simulink model "untitled (2)"  (R2020a)
settings: Solver=VariableStepAuto  StartTime=0.0  StopTime=3  RelTol=1e-3
libraries: simulink x1
settings Model: Creator=nose  LastModifiedBy=nose

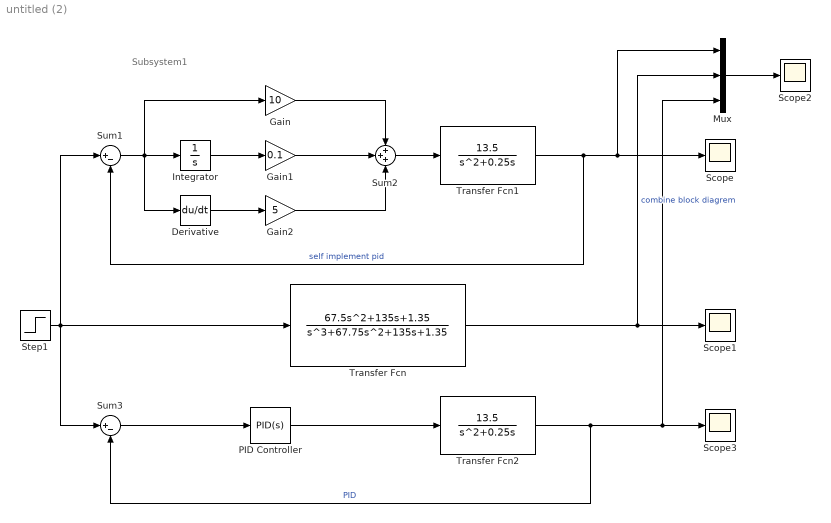
== system untitled (2) ==
  note: Subsystem1
  Derivative : Derivative
  Gain : Gain  Gain=10
  Gain1 : Gain  Gain=0.1
  Gain2 : Gain  Gain=5
  Integrator : Integrator
  Mux : Mux  Inputs=3
  PID Controller : simulink/Continuous/PID Controller  Controller=PID  Form=Parallel  TimeDomain=Continuous-time  UseExternalTs=off  SampleTime=-1  IntegratorMethod=Forward Euler  FilterMethod=Forward Euler  ControllerParametersSource=internal  P=10  I=0.1  D=5  UseFilter=on  N=100  TunerSelectOption=Transfer Function Based (PID Tuner App)  InitialConditionSource=internal  InitialConditionForIntegrator=0  InitialConditionForFilter=0  DifferentiatorICPrevScaledInput=0  ExternalReset=none  TrackingMode=off  Kt=1  LimitOutput=off  UpperSaturationLimit=inf  LowerSaturationLimit=-inf  LinearizeAsGain=on  AntiWindupMode=none  Kb=1  POutMin=[]  POutMax=[]  IOutMin=[]  IOutMax=[]  DOutMin=[]  DOutMax=[]  NOutMin=[]  NOutMax=[]  SumOutMin=[]  SumOutMax=[]  SaturationOutMin=[]  SaturationOutMax=[]  PParamMin=[]  PParamMax=[]  IParamMin=[]  IParamMax=[]  DParamMin=[]  DParamMax=[]  NParamMin=[]  NParamMax=[]  KbParamMin=[]  KbParamMax=[]  KtParamMin=[]  KtParamMax=[]  KbOutMin=[]  KbOutMax=[]  KtOutMin=[]  KtOutMax=[]  IntegratorOutMin=[]  IntegratorOutMax=[]  FilterOutMin=[]  FilterOutMax=[]  SumI1OutMin=[]  SumI1OutMax=[]  SumI2OutMin=[]  SumI2OutMax=[]  SumI3OutMin=[]  SumI3OutMax=[]  SumI4OutMin=[]  SumI4OutMax=[]  SumDOutMin=[]  SumDOutMax=[]  DifferentiatorOutMin=[]  DifferentiatorOutMax=[]  FilterDiffOutCoefMin=[]  FilterDiffOutCoefMax=[]  ReciprocalOutMin=[]  ReciprocalOutMax=[]  SumDenOutMin=[]  SumDenOutMax=[]  SumNumOutMin=[]  SumNumOutMax=[]  DivideOutMin=[]  DivideOutMax=[]  UdiffTsProdOutMin=[]  UdiffTsProdOutMax=[]  NTsProdOutMin=[]  NTsProdOutMax=[]  UintegralTsProdOutMin=[]  UintegralTsProdOutMax=[]  UngainTsProdOutMin=[]  UngainTsProdOutMax=[]  IntegratorContinuousStateAttributes=''  IntegratorStateMustResolveToSignalObject=off  IntegratorRTWStateStorageClass=Auto  FilterContinuousStateAttributes=''  FilterStateMustResolveToSignalObject=off  FilterRTWStateStorageClass=Auto  ParallelPVariant=InternalParameters  IdealPVariant=Disabled  IVariant=InternalParameters  DVariant=InternalParameters  IntegratorVariant=Continuous  SatVariant=Disabled  AWVariant=Passthrough  PCopyVariant=Disabled  TRVariant=Disabled  FdbkBlocksVariant=Forward  IdealPFdbkVariant=Disabled  SatFdbkVariant=Disabled  DerivativeFilterVariant=ContFilter  NVariant=InternalParameters  NCopyVariant=Disabled  FilterICVariant=InternalICsFilter  IntegratorICVariant=InternalICs  ExternalResetVariant=Disabled  TRSumVariant=Passthrough  SumFdbkVariant=Disabled  SumVariant=Sum_PID  TsampFilterVariant=InternalTs  TsampNgainVariant=Passthrough  TsampIntegralVariant=Passthrough
  Scope{,1..3} (4 alike) : Scope
  Step1 : Step  SampleTime=0  ZeroCross=off
  Sum1 : Sum  Inputs=|+-
  Sum2 : Sum  Inputs=+++
  Sum3 : Sum  Inputs=|+-
  Transfer Fcn : TransferFcn  Numerator=[67.5 135 1.35]  Denominator=[1 67.75 135 1.35]
  Transfer Fcn1 : TransferFcn  Numerator=[13.5]  Denominator=[1 0.25 0]
  Transfer Fcn2 : TransferFcn  Numerator=[13.5]  Denominator=[1 0.25 0]
  wires:
  Transfer Fcn1/1 -> Sum1/2, Scope/1, Mux/1  "self implement pid"
  Gain2/1 -> Sum2/3
  Gain1/1 -> Sum2/2
  Derivative/1 -> Gain2/1
  Integrator/1 -> Gain1/1
  Sum1/1 -> Derivative/1, Gain/1, Integrator/1
  Gain/1 -> Sum2/1
  Step1/1 -> Sum1/1, Sum3/1, Transfer Fcn/1
  Transfer Fcn/1 -> Scope1/1, Mux/2  "combine block diagrem"
  Sum2/1 -> Transfer Fcn1/1
  PID Controller/1 -> Transfer Fcn2/1
  Transfer Fcn2/1 -> Scope3/1, Mux/3, Sum3/2  "PID"
  Sum3/1 -> PID Controller/1
  Mux/1 -> Scope2/1
